simulink model "q10"  (R2020b)
settings: Solver=VariableStepAuto  StartTime=0.0  StopTime=100  RelTol=1e-3
values from neighbouring files (symbols this model uses):
  A = 15.5179    [l3q6.m]
  constant = (2*a^2*g)^0.5 / Km    (= 2.03217090667)    [l3q6.m]
  L0 = 15    [l3q6.m]
settings Model: Creator=thaibinhbr97  LastModifiedBy=thaibinhbr97

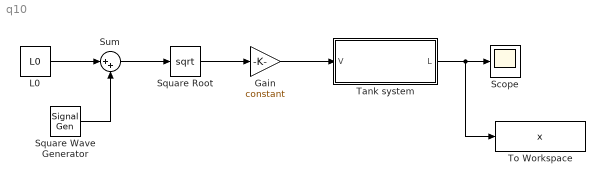
== system q10 ==
  Gain : Gain  Gain=constant
  L0 : Constant  Value=L0
  Scope : Scope
  Square Root : Sqrt  SaturateOnIntegerOverflow=on
  Square Wave Generator : SignalGenerator  WaveForm=square  Frequency=0.1
  Sum : Sum  Inputs=|++
  Tank system : Subsystem
  To Workspace : ToWorkspace  VariableName=x  SaveFormat=Timeseries  SampleTime=-1
  wires:
  Tank system/1(L) -> To Workspace/1, Scope/1
  Square Root/1 -> Gain/1
  Gain/1 -> Tank system/1(V)
  Square Wave Generator/1 -> Sum/2
  L0/1 -> Sum/1
  Sum/1 -> Square Root/1

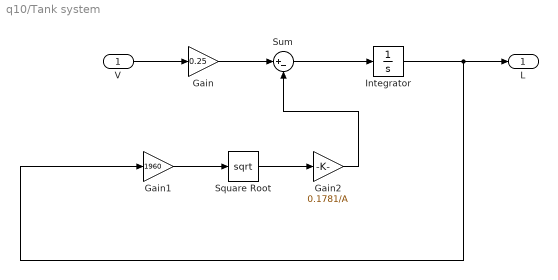
== system q10/Tank system ==
  V : Inport
  Gain : Gain  Gain=0.25
  Gain1 : Gain  Gain=1960
  Gain2 : Gain  Gain=0.1781/A
  Integrator : Integrator
  Square Root : Sqrt  SaturateOnIntegerOverflow=on
  Sum : Sum  Inputs=|+-
  L : Outport
  wires:
  V/1 -> Gain/1
  Gain/1 -> Sum/1
  Sum/1 -> Integrator/1
  Integrator/1 -> Gain1/1, L/1
  Square Root/1 -> Gain2/1
  Gain1/1 -> Square Root/1
  Gain2/1 -> Sum/2
